simulink library "find6DOFSnellMin9_cl"  (R2018b)
settings: Solver=VariableStepAuto  StartTime=0.0  StopTime=10.0  RelTol=1e-3
undefined symbols (not defined in the file or in its folder): params, snells
libraries: rayTrace_ul x9, powellsMethodMin_ul x1
settings Model: Creator=MAE-NCSUCORE  LastModifiedBy=MAE-NCSUCORE

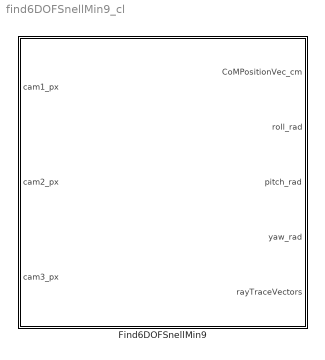
== system find6DOFSnellMin9_cl ==
  Find6DOFSnellMin9 : Subsystem  mask{imageDims_px=params.sideImageSize_px.Value, initialCoMPositionVec_cm=params.initCoMPosVec_cm.Value, initialEulerAngles_deg=params.initEulerAng_deg.Value, indxOfRefVec=params.indexOfRefractionA.Value, glassThickness_cm=params.glassThickness_cm.Value, snells=snells, glassPlane=1, cameraFOVAngles_deg=params.cameraFOV_deg.Value, sideEulerAngles_deg=params.sideCamEulAng_deg.Value, sideCamPositionVec_cm=params.sideCamPosVec_cm.Value, sideCamDistToGlass_cm=params.sideDistancetoGlass_cm.Value, botEulerAngles_deg=params.botCamEulAng_deg.Value, botCamPositionVec_cm=params.botCamPosVec_cm.Value, botCamDistToGlass_cm=params.botDistancetoGlass_cm.Value, slantEulerAngles_deg=params.slntCamEulAng_deg.Value, slantCamPositionVec_cm=params.slntCamPosVec_cm.Value, slantCamDistToGlass_cm=params.slntDistancetoGlass_cm.Value, sideSeparation_cm=params.sideDotSepDist_cm.Value, sidePositionVecBF_cm=params.sideDotPosVec_cm.Value, bottomASeparation_cm=params.botADotSepDist_cm.Value, botAPositionVecBF_cm=params.botADotPosVec_cm.Value, bottomBSeparation_cm=params.botBDotSepDist_cm.Value, botBPositionVecBF_cm=params.botBDotPosVec_cm.Value}
      mask prompts: imageDims_px "Image Dimensions [rows, cols] [px]"; initialCoMPositionVec_cm "Initial CoM Position Vector [cm]"; initialEulerAngles_deg "Initial Euler Angles [deg]"; indxOfRefVec "Indices of Refraction, [air glass water]"; glassThickness_cm "Glass Thickness [cm]"; snells "Snells Parameter Structure"; glassPlane "Glass Plane (1 = xy, 2 = xz)"; cameraFOVAngles_deg "Field of View Angles [horiz, vert] [deg]"; sideEulerAngles_deg "Euler Angles [roll pitch yaw] [deg]"; sideCamPositionVec_cm "Position Vector [cm]"; sideCamDistToGlass_cm "Distance to Glass [cm]"; botEulerAngles_deg "Euler Angles [roll pitch yaw]  [deg]"; botCamPositionVec_cm "Position Vector [cm]"; botCamDistToGlass_cm "Distance to Glass [cm]"; slantEulerAngles_deg "Euler Angles [roll pitch yaw]  [deg]"; slantCamPositionVec_cm "Position Vec [cm]"; slantCamDistToGlass_cm "Distance to Glass [cm]"; sideSeparation_cm "Separation Distance [cm]"; sidePositionVecBF_cm "Centroid Position in Body Frame [cm]"; bottomASeparation_cm "Separation Distance [cm]"; botAPositionVecBF_cm "Centroid Position in Body Frame [cm]"; bottomBSeparation_cm "Separation Distance [cm]"; botBPositionVecBF_cm "Centroid Position in Body Frame [cm]"
      mask init:
      | find6DOFSnellMin_init;
      mask DialogControl Container4 Prompt: Camera Properties
      mask DialogControl Container7 Prompt: Side Camera
      mask DialogControl Container8 Prompt: Bottom Camera
      mask DialogControl Container9 Prompt: Slant Camera
      mask DialogControl Container13 Prompt: Dot Properties
      mask DialogControl Container14 Prompt: Side Dots
      mask DialogControl Container15 Prompt: Bottom Dot Set A
      mask DialogControl Container16 Prompt: Bottom Dot Set B
      mask Display:
      | image('blockImage.png',[.2, .2, .6, .6],'on');
      | 
      | port_label('input',1,'Camera 1')
      | port_label('input',2,'Camera 2')
      | port_label('input',3,'Camera 3')
      | 
      | port_label('output',1,'CoMPosVec_cm')
      | port_label('output',2,'roll_rad')
      | port_label('output',3,'pitch_rad')
      | port_label('output',4,'yaw_rad')
      | port_label('output',5,'rayTraceVec')
      | 
      | % port_label('output',5,'rxRaw')
      | % port_label('output',6,'ryRaw')
      | 
      | text(0.5, 1, 'Snells Law - Resolve 6 DOF', 'horizontalAlignment', 'center', ...
      |   'verticalAlignment', 'top')

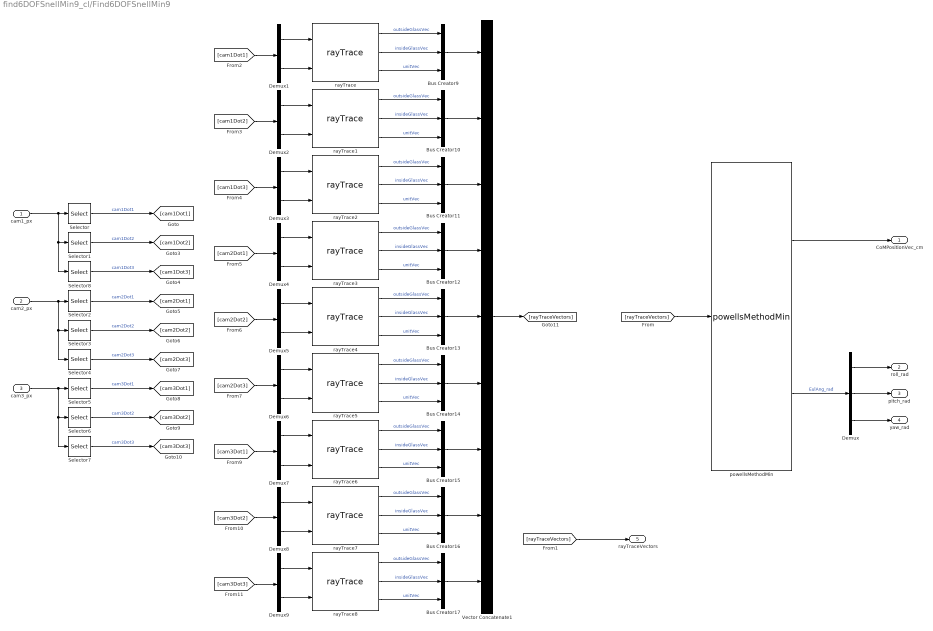
== system find6DOFSnellMin9_cl/Find6DOFSnellMin9 ==
  cam1_px : Inport
  cam2_px : Inport  Port=2
  cam3_px : Inport  Port=3
  Bus Creator{9..17} (9 alike) : BusCreator  Inputs=3  OutDataTypeStr=Bus: rayBus  NonVirtualBus=on
  Demux : Demux  Outputs=3
  Demux{1..9} (9 alike) : Demux  Outputs=2
  Selector : Selector  InputPortWidth=6  IndexOptions=Index vector (dialog)  Indices=[1 2]  OutputSizes=1
  Selector1 : Selector  InputPortWidth=6  IndexOptions=Index vector (dialog)  Indices=[3 4]  OutputSizes=1
  Selector2 : Selector  InputPortWidth=6  IndexOptions=Index vector (dialog)  Indices=[1 2]  OutputSizes=1
  Selector3 : Selector  InputPortWidth=6  IndexOptions=Index vector (dialog)  Indices=[3 4]  OutputSizes=1
  Selector4 : Selector  InputPortWidth=6  IndexOptions=Index vector (dialog)  Indices=[5 6]  OutputSizes=1
  Selector5 : Selector  InputPortWidth=6  IndexOptions=Index vector (dialog)  Indices=[1 2]  OutputSizes=1
  Selector6 : Selector  InputPortWidth=6  IndexOptions=Index vector (dialog)  Indices=[3 4]  OutputSizes=1
  Selector7 : Selector  InputPortWidth=6  IndexOptions=Index vector (dialog)  Indices=[5 6]  OutputSizes=1
  Selector8 : Selector  InputPortWidth=6  IndexOptions=Index vector (dialog)  Indices=[5 6]  OutputSizes=1
  Vector Concatenate1 : Concatenate  NumInputs=9
  powellsMethodMin : powellsMethodMin_ul/powellsMethodMin  initialEulerAngles_rad=initialEulerAngles_rad  snells=snells
  rayTrace : rayTrace_ul/rayTrace  camPosVec_cm=snells(1).camPosVec  camEulAngles_deg=snells(1).camEulAng  dist2Glass_cm=snells(1).camDist2Glass  indOfRefVec=indxOfRefVec  glassPlane=glassPlane  glassThickness_cm=glassThickness_cm  imageDimsVec_px=imageDims_px  camFOV_deg=cameraFOVAngles_deg
  rayTrace1 : rayTrace_ul/rayTrace  camPosVec_cm=snells(2).camPosVec  camEulAngles_deg=snells(2).camEulAng  dist2Glass_cm=snells(2).camDist2Glass  indOfRefVec=indxOfRefVec  glassPlane=glassPlane  glassThickness_cm=glassThickness_cm  imageDimsVec_px=imageDims_px  camFOV_deg=cameraFOVAngles_deg
  rayTrace2 : rayTrace_ul/rayTrace  camPosVec_cm=snells(3).camPosVec  camEulAngles_deg=snells(3).camEulAng  dist2Glass_cm=snells(3).camDist2Glass  indOfRefVec=indxOfRefVec  glassPlane=glassPlane  glassThickness_cm=glassThickness_cm  imageDimsVec_px=imageDims_px  camFOV_deg=cameraFOVAngles_deg
  rayTrace3 : rayTrace_ul/rayTrace  camPosVec_cm=snells(4).camPosVec  camEulAngles_deg=snells(4).camEulAng  dist2Glass_cm=snells(4).camDist2Glass  indOfRefVec=indxOfRefVec  glassPlane=glassPlane  glassThickness_cm=glassThickness_cm  imageDimsVec_px=imageDims_px  camFOV_deg=cameraFOVAngles_deg
  rayTrace4 : rayTrace_ul/rayTrace  camPosVec_cm=snells(5).camPosVec  camEulAngles_deg=snells(5).camEulAng  dist2Glass_cm=snells(5).camDist2Glass  indOfRefVec=indxOfRefVec  glassPlane=glassPlane  glassThickness_cm=glassThickness_cm  imageDimsVec_px=imageDims_px  camFOV_deg=cameraFOVAngles_deg
  rayTrace5 : rayTrace_ul/rayTrace  camPosVec_cm=snells(6).camPosVec  camEulAngles_deg=snells(6).camEulAng  dist2Glass_cm=snells(6).camDist2Glass  indOfRefVec=indxOfRefVec  glassPlane=glassPlane  glassThickness_cm=glassThickness_cm  imageDimsVec_px=imageDims_px  camFOV_deg=cameraFOVAngles_deg
  rayTrace6 : rayTrace_ul/rayTrace  camPosVec_cm=snells(7).camPosVec  camEulAngles_deg=snells(7).camEulAng  dist2Glass_cm=snells(7).camDist2Glass  indOfRefVec=indxOfRefVec  glassPlane=glassPlane  glassThickness_cm=glassThickness_cm  imageDimsVec_px=imageDims_px  camFOV_deg=cameraFOVAngles_deg
  rayTrace7 : rayTrace_ul/rayTrace  camPosVec_cm=snells(8).camPosVec  camEulAngles_deg=snells(8).camEulAng  dist2Glass_cm=snells(8).camDist2Glass  indOfRefVec=indxOfRefVec  glassPlane=glassPlane  glassThickness_cm=glassThickness_cm  imageDimsVec_px=imageDims_px  camFOV_deg=cameraFOVAngles_deg
  rayTrace8 : rayTrace_ul/rayTrace  camPosVec_cm=snells(9).camPosVec  camEulAngles_deg=snells(9).camEulAng  dist2Glass_cm=snells(9).camDist2Glass  indOfRefVec=indxOfRefVec  glassPlane=glassPlane  glassThickness_cm=glassThickness_cm  imageDimsVec_px=imageDims_px  camFOV_deg=cameraFOVAngles_deg
  CoMPositionVec_cm : Outport
  roll_rad : Outport  Port=2
  pitch_rad : Outport  Port=3
  yaw_rad : Outport  Port=4
  rayTraceVectors : Outport  Port=5
  wires:
  powellsMethodMin/1 -> CoMPositionVec_cm/1
  powellsMethodMin/2 -> Demux/1  "EulAng_rad"
  Demux/1 -> roll_rad/1
  Demux/3 -> yaw_rad/1
  Demux/2 -> pitch_rad/1
  cam1_px/1 -> Selector/1, Selector1/1, Selector8/1
  cam2_px/1 -> Selector4/1, Selector3/1, Selector2/1
  cam3_px/1 -> Selector5/1, Selector6/1, Selector7/1
  [rayTraceVectors] -> powellsMethodMin/1
  Selector/1 -> [cam1Dot1]  "cam1Dot1"
  Selector1/1 -> [cam1Dot2]  "cam1Dot2"
  Selector8/1 -> [cam1Dot3]  "cam1Dot3"
  Selector2/1 -> [cam2Dot1]  "cam2Dot1"
  Selector3/1 -> [cam2Dot2]  "cam2Dot2"
  Selector4/1 -> [cam2Dot3]  "cam2Dot3"
  Selector5/1 -> [cam3Dot1]  "cam3Dot1"
  Selector6/1 -> [cam3Dot2]  "cam3Dot2"
  Selector7/1 -> [cam3Dot3]  "cam3Dot3"
  Demux1/2 -> rayTrace/2
  Demux1/1 -> rayTrace/1
  Demux2/2 -> rayTrace1/2
  Demux2/1 -> rayTrace1/1
  Demux3/2 -> rayTrace2/2
  Demux3/1 -> rayTrace2/1
  Demux4/1 -> rayTrace3/1
  Demux4/2 -> rayTrace3/2
  Demux5/1 -> rayTrace4/1
  Demux5/2 -> rayTrace4/2
  Demux6/1 -> rayTrace5/1
  Demux6/2 -> rayTrace5/2
  Demux7/1 -> rayTrace6/1
  Demux7/2 -> rayTrace6/2
  Demux8/1 -> rayTrace7/1
  Demux8/2 -> rayTrace7/2
  Demux9/1 -> rayTrace8/1
  Demux9/2 -> rayTrace8/2
  [cam1Dot1] -> Demux1/1
  [cam1Dot2] -> Demux2/1
  [cam1Dot3] -> Demux3/1
  [cam2Dot1] -> Demux4/1
  [cam2Dot2] -> Demux5/1
  [cam2Dot3] -> Demux6/1
  [cam3Dot1] -> Demux7/1
  [cam3Dot2] -> Demux8/1
  [cam3Dot3] -> Demux9/1
  rayTrace/3 -> Bus Creator9/3  "unitVec"
  rayTrace/2 -> Bus Creator9/2  "insideGlassVec"
  rayTrace/1 -> Bus Creator9/1  "outsideGlassVec"
  rayTrace1/1 -> Bus Creator10/1  "outsideGlassVec"
  rayTrace1/2 -> Bus Creator10/2  "insideGlassVec"
  rayTrace1/3 -> Bus Creator10/3  "unitVec"
  rayTrace8/3 -> Bus Creator17/3  "unitVec"
  rayTrace8/2 -> Bus Creator17/2  "insideGlassVec"
  rayTrace8/1 -> Bus Creator17/1  "outsideGlassVec"
  rayTrace7/3 -> Bus Creator16/3  "unitVec"
  rayTrace7/2 -> Bus Creator16/2  "insideGlassVec"
  rayTrace7/1 -> Bus Creator16/1  "outsideGlassVec"
  rayTrace6/3 -> Bus Creator15/3  "unitVec"
  rayTrace6/2 -> Bus Creator15/2  "insideGlassVec"
  rayTrace6/1 -> Bus Creator15/1  "outsideGlassVec"
  rayTrace5/3 -> Bus Creator14/3  "unitVec"
  rayTrace5/2 -> Bus Creator14/2  "insideGlassVec"
  rayTrace5/1 -> Bus Creator14/1  "outsideGlassVec"
  rayTrace4/3 -> Bus Creator13/3  "unitVec"
  rayTrace4/2 -> Bus Creator13/2  "insideGlassVec"
  rayTrace4/1 -> Bus Creator13/1  "outsideGlassVec"
  rayTrace3/3 -> Bus Creator12/3  "unitVec"
  rayTrace3/2 -> Bus Creator12/2  "insideGlassVec"
  rayTrace3/1 -> Bus Creator12/1  "outsideGlassVec"
  rayTrace2/3 -> Bus Creator11/3  "unitVec"
  rayTrace2/2 -> Bus Creator11/2  "insideGlassVec"
  rayTrace2/1 -> Bus Creator11/1  "outsideGlassVec"
  Bus Creator9/1 -> Vector Concatenate1/1
  Bus Creator10/1 -> Vector Concatenate1/2
  Bus Creator11/1 -> Vector Concatenate1/3
  Bus Creator12/1 -> Vector Concatenate1/4
  Bus Creator13/1 -> Vector Concatenate1/5
  Bus Creator14/1 -> Vector Concatenate1/6
  Bus Creator15/1 -> Vector Concatenate1/7
  Bus Creator16/1 -> Vector Concatenate1/8
  Bus Creator17/1 -> Vector Concatenate1/9
  Vector Concatenate1/1 -> [rayTraceVectors]
  [rayTraceVectors] -> rayTraceVectors/1
